simulink model "LAB1_Signals"  (R2020b)
settings: Solver=VariableStepAuto  StartTime=0.0  StopTime=10.0  RelTol=1e-3
settings Model: Creator=dssan  LastModifiedBy=dssan

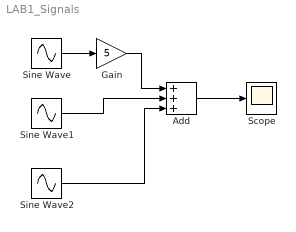
== system LAB1_Signals ==
  Add : Sum  Inputs=+++
  Gain : Gain  Gain=5
  Scope : Scope
  Sine Wave : Sin  SampleTime=0
  Sine Wave1 : Sin  Frequency=10  SampleTime=0
  Sine Wave2 : Sin  Amplitude=0.5  Frequency=100  SampleTime=0
  wires:
  Add/1 -> Scope/1
  Sine Wave/1 -> Gain/1
  Sine Wave1/1 -> Add/2
  Gain/1 -> Add/1
  Sine Wave2/1 -> Add/3
